simulink model "w13_OOP"  (R2025a)
settings: Solver=VariableStepAuto  StartTime=0.0  StopTime=inf  FixedStep=1e-5  MaxStep=1e-4  RelTol=1e-3
values from neighbouring files (symbols this model uses):
  B = 0.0001    [main.m]
  J = 0.045    [main.m]
  Kic = Rs*Wcc    (= 1256.63706144)    [main.m]
  Kpc = Lds*Wcc    (= 18.8495559215)    [main.m]
  Lamf = 0.12    [main.m]
  Lds = 30.0e-3    (= 0.03)    [main.m]
  Lqs = 40.0e-3    (= 0.04)    [main.m]
  P = 24    [main.m]
  Rs = 2    [main.m]
  V_inj = 60    [main.m]
  w_h = 2*pi*1000    (= 6283.18530718)    [main.m]
settings Model: Creator=moon  LastModifiedBy=mun97
settings RTWCC: GPUComputeCapability=3.5

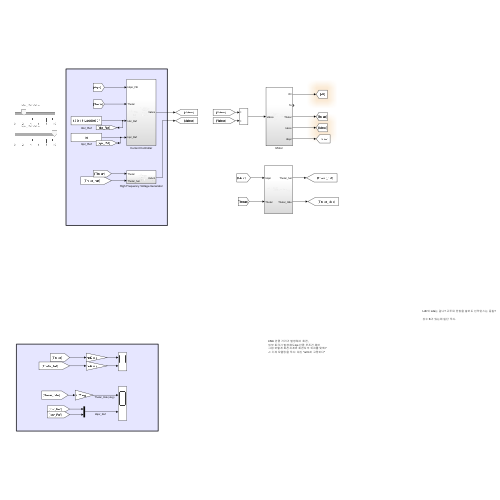
[thumbnail: Simulink's stored preview of the top-level diagram]
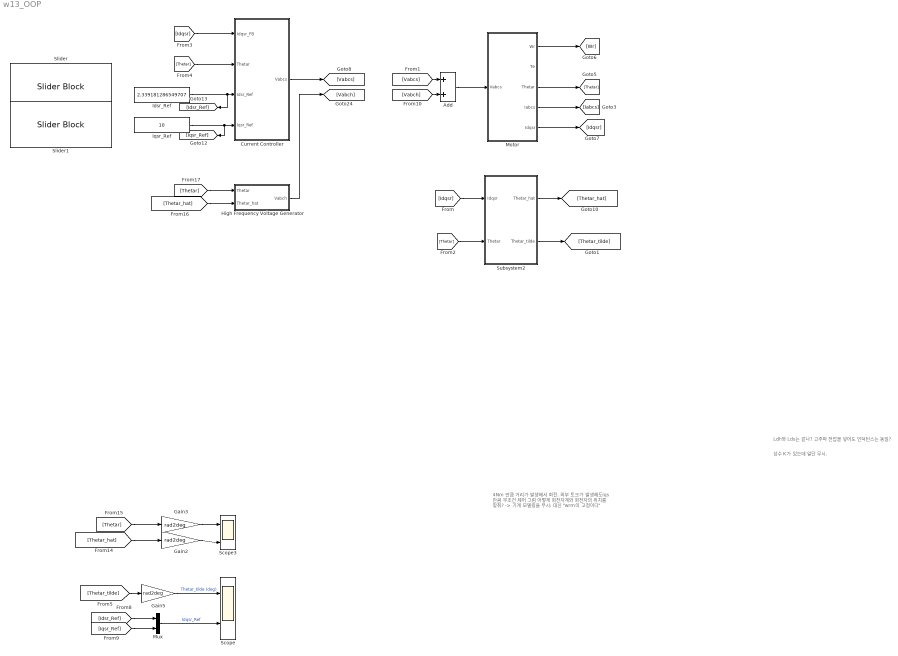
== system w13_OOP ==
  note: Ldh와 Lds는 같나? 고주파 전압을 넣어도 인덕턴스는 동일?
  note: 4Nm 만큼 거리가 발생해서 회전,
      | 외부 토크가 발생해도iqs 만큼 무조건 제어
      | 그럼 어떻게 회전자계와 회전자의 위치를 맞춰?
      | -> 기계 모델링을 무시: 대신 "wrm이 고정이다"
  note: 상수 K가 있는데 일단 무시.
  Add : Sum
  Current Controller : Subsystem
  Gain2 : Gain  Gain=rad2deg
  Gain3 : Gain  Gain=rad2deg
  Gain5 : Gain  Gain=rad2deg
  High Frequency Voltage Generator : Subsystem
  Idsr_Ref : Constant  Value=2.339181286549707
  Iqsr_Ref : Constant  Value=10
  Motor : Subsystem
  Mux : Mux  Inputs=2
  Scope : Scope  NumInputPorts=2
      settings: ActiveDisplayYMinimum=-68.281824450280524  ActiveDisplayYMaximum=129.406425416175  DataLoggingVariableName=ScopeData8
  Scope3 : Scope  NumInputPorts=2
      settings: ActiveDisplayYMinimum=-77.2256556656794  ActiveDisplayYMaximum=78.097651862279335  DataLoggingVariableName=ScopeData11
  Slider : SliderBlock  ScaleMax=10
  Slider1 : SliderBlock  ScaleMax=10
  Subsystem2 : Subsystem
  wires:
  Motor/4(Iabcs) -> [Iabcs]
  Motor/3(Thetar) -> [Thetar]
  Motor/1(Wr) -> [Wr]
  Motor/5(Idqsr) -> [Idqsr]
  [Idqsr] -> Current Controller/1(Idqsr_FB)
  Current Controller/1(Vabcs) -> [Vabcs]
  [Thetar] -> Current Controller/2(Thetar)
  Idsr_Ref/1 -> [Idsr_Ref], Current Controller/3(Idsr_Ref)
  Iqsr_Ref/1 -> Current Controller/4(Iqsr_Ref), [Iqsr_Ref]
  [Vabcs] -> Add/1
  [Vabch] -> Add/2
  Add/1 -> Motor/1(Vabcs)
  [Thetar] -> Gain3/1
  [Thetar_hat] -> Gain2/1
  Gain2/1 -> Scope3/2
  Gain3/1 -> Scope3/1
  Gain5/1 -> Scope/1  "Thetar_tilde (deg)"
  [Thetar_tilde] -> Gain5/1
  [Idsr_Ref] -> Mux/1
  [Iqsr_Ref] -> Mux/2
  Mux/1 -> Scope/2  "Idqsr_Ref"
  High Frequency Voltage Generator/1(Vabch) -> [Vabch]
  [Thetar] -> High Frequency Voltage Generator/1(Thetar)
  [Thetar_hat] -> High Frequency Voltage Generator/2(Thetar_hat)
  [Idqsr] -> Subsystem2/1(Idqsr)
  [Thetar] -> Subsystem2/2(Thetar)
  Subsystem2/1(Thetar_hat) -> [Thetar_hat]
  Subsystem2/2(Thetar_tilde) -> [Thetar_tilde]

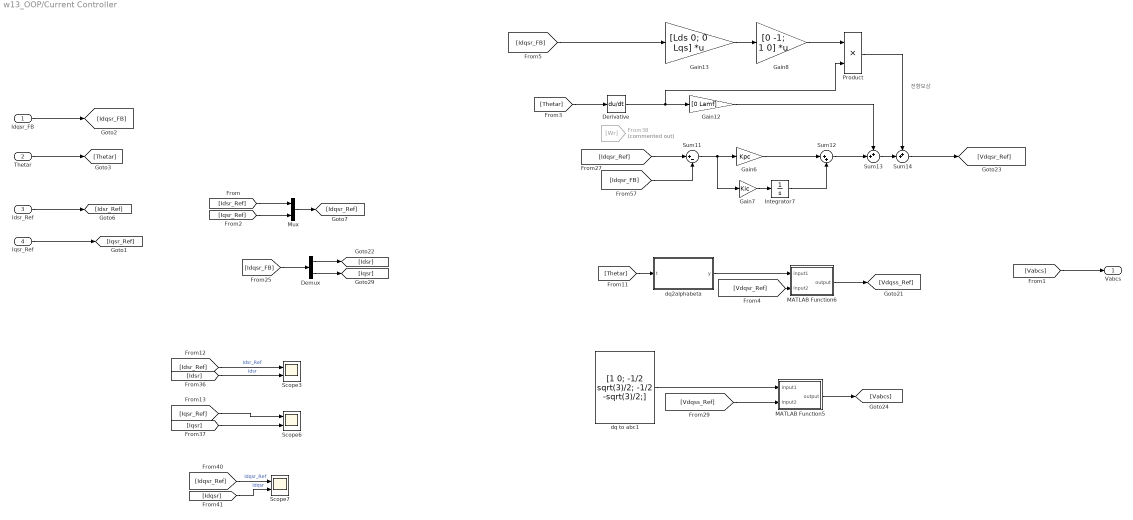
== system w13_OOP/Current Controller ==
  note: 전향보상
  Idqsr_FB : Inport
  Thetar : Inport  Port=2
  Idsr_Ref : Inport  Port=3
  Iqsr_Ref : Inport  Port=4
  Demux : Demux  Outputs=2
  Derivative : Derivative
  From38 : From  Commented=on  GotoTag=Wr
  Gain12 : Gain  Gain=[0 Lamf]
  Gain13 : Gain  Gain=[Lds 0; 0 Lqs]  Multiplication=Matrix(K*u)
  Gain6 : Gain  Gain=Kpc
  Gain7 : Gain  Gain=Kic
  Gain8 : Gain  Gain=[0 -1; 1 0]  Multiplication=Matrix(K*u)
  Integrator7 : Integrator
  MATLAB Function5 : MATLAB Function  TreatAsAtomicUnit=on
  MATLAB Function6 : MATLAB Function  TreatAsAtomicUnit=on
  Mux : Mux  Inputs=2
  Product : Product
  Scope3 : Scope  NumInputPorts=2
      settings: ActiveDisplayYMinimum=-5.30172  ActiveDisplayYMaximum=0.86593  DataLoggingVariableName=ScopeData4
  Scope6 : Scope  NumInputPorts=2
      settings: ActiveDisplayYMinimum=-0.50888  ActiveDisplayYMaximum=4.57994  DataLoggingVariableName=ScopeData5
  Scope7 : Scope  NumInputPorts=2
      settings: ActiveDisplayYMinimum=-5.25048  ActiveDisplayYMaximum=7.25433  DataLoggingVariableName=ScopeData6
  Sum11 : Sum  Inputs=|+-
  Sum12 : Sum  Inputs=|++
  Sum13 : Sum  Inputs=++|
  Sum14 : Sum  Inputs=++|
  dq to abc1 : Constant  Value=[1 0; -1/2 sqrt(3)/2; -1/2 -sqrt(3)/2;]
      mask Display: image(imread('img/dq2abc.png'))
  dq2alphabeta : Subsystem
      mask Display: image(imread('img/rotateMatrix.png'))
  Vabcs : Outport
  wires:
  [Vdqss_Ref] -> MATLAB Function5/2(input2)
  Product/1 -> Sum14/1
  [Thetar] -> dq2alphabeta/1(t)
  [Idqsr] -> Scope7/2  "Idqsr"
  Idsr_Ref/1 -> [Idsr_Ref]
  [Idqsr_FB] -> Gain13/1
  [Iqsr_Ref] -> Scope6/1
  dq2alphabeta/1(y) -> MATLAB Function6/1(input1)
  [Idqsr_Ref] -> Scope7/1  "Idqsr_Ref"
  Demux/2 -> [Iqsr]
  Gain13/1 -> Gain8/1
  [Idsr] -> Scope3/2  "Idsr"
  MATLAB Function6/1(output) -> [Vdqss_Ref]
  Sum14/1 -> [Vdqsr_Ref]
  Sum13/1 -> Sum14/2
  dq to abc1/1 -> MATLAB Function5/1(input1)
  Demux/1 -> [Idsr]
  [Idqsr_FB] -> Sum11/2
  Integrator7/1 -> Sum12/2
  Gain8/1 -> Product/1
  [Idsr_Ref] -> Scope3/1  "Idsr_Ref"
  Gain6/1 -> Sum12/1
  Derivative/1 -> Product/2, Gain12/1
  [Idqsr_Ref] -> Sum11/1
  MATLAB Function5/1(output) -> [Vabcs]
  [Iqsr] -> Scope6/2
  Gain12/1 -> Sum13/1
  [Idqsr_FB] -> Demux/1
  Sum11/1 -> Gain7/1, Gain6/1
  [Vdqsr_Ref] -> MATLAB Function6/2(input2)
  Sum12/1 -> Sum13/2
  Gain7/1 -> Integrator7/1
  Idqsr_FB/1 -> [Idqsr_FB]
  [Vabcs] -> Vabcs/1
  Thetar/1 -> [Thetar]
  Iqsr_Ref/1 -> [Iqsr_Ref]
  [Idsr_Ref] -> Mux/1
  Mux/1 -> [Idqsr_Ref]
  [Iqsr_Ref] -> Mux/2
  [Thetar] -> Derivative/1

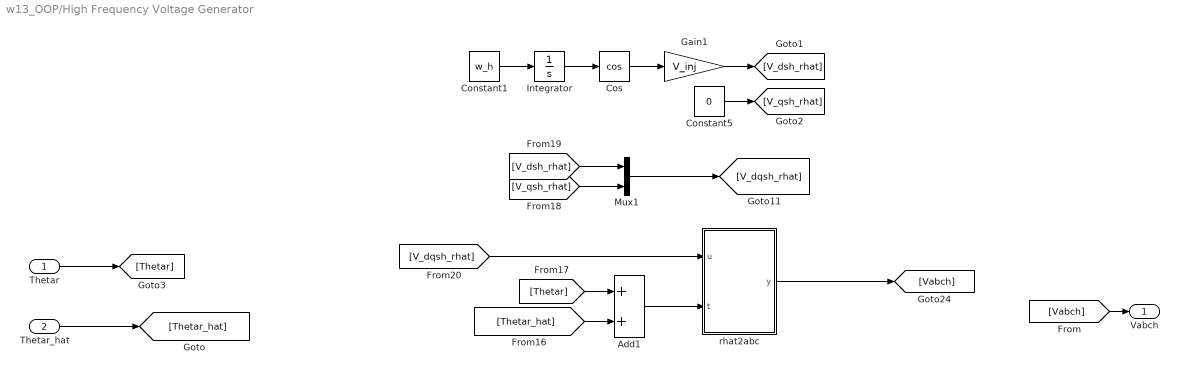
== system w13_OOP/High Frequency Voltage Generator ==
  Thetar : Inport
  Thetar_hat : Inport  Port=2
  Add1 : Sum
  Constant1 : Constant  Value=w_h
  Constant5 : Constant  Value=0
  Cos : Trigonometry  Operator=cos
  Gain1 : Gain  Gain=V_inj
  Integrator : Integrator
  Mux1 : Mux  Inputs=2
  rhat2abc : MATLAB Function  TreatAsAtomicUnit=on
  Vabch : Outport
  wires:
  Constant5/1 -> [V_qsh_rhat]
  Integrator/1 -> Cos/1
  Constant1/1 -> Integrator/1
  Mux1/1 -> [V_dqsh_rhat]
  Gain1/1 -> [V_dsh_rhat]
  rhat2abc/1(y) -> [Vabch]
  Add1/1 -> rhat2abc/2(t)
  Cos/1 -> Gain1/1
  [V_dsh_rhat] -> Mux1/1
  [V_qsh_rhat] -> Mux1/2
  [Thetar_hat] -> Add1/2
  [Thetar] -> Add1/1
  [V_dqsh_rhat] -> rhat2abc/1(u)
  [Vabch] -> Vabch/1
  Thetar_hat/1 -> [Thetar_hat]
  Thetar/1 -> [Thetar]

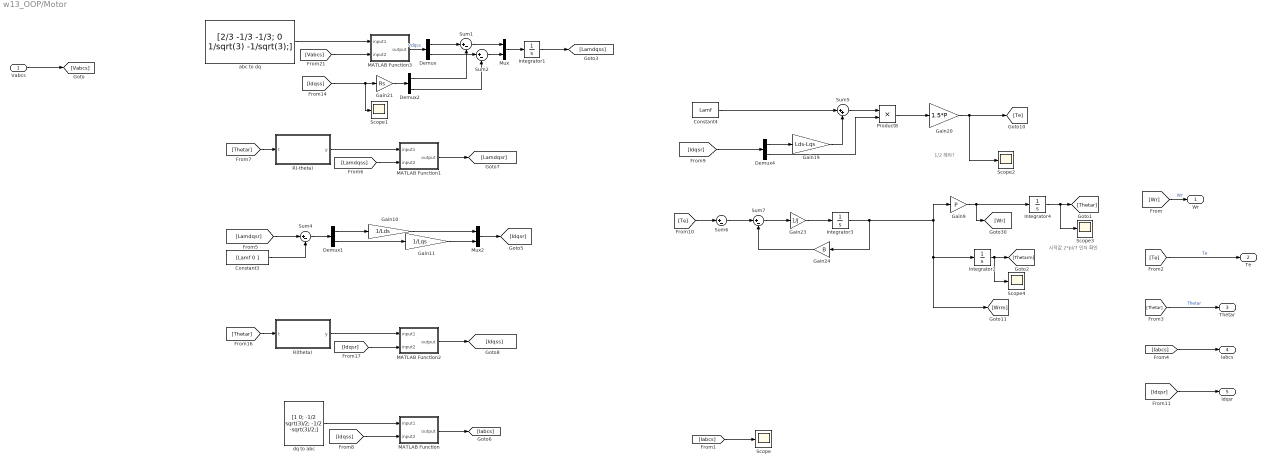
== system w13_OOP/Motor ==
  note: 시작값 2*pi/7 인지 확인
  note: 1/2 해야?
  Vabcs : Inport
  Constant3 : Constant  Value=[Lamf 0 ]
  Constant4 : Constant  Value=Lamf
  Demux{,1..2,4} (4 alike) : Demux  Outputs=2
  Gain10 : Gain  Gain=1/Lds
  Gain11 : Gain  Gain=1/Lqs
  Gain19 : Gain  Gain=Lds-Lqs
  Gain20 : Gain  Gain=1.5*P
  Gain21 : Gain  Gain=Rs
  Gain23 : Gain  Gain=1/J
  Gain24 : Gain  Gain=B
  Gain9 : Gain  Gain=P
  Integrator1 : Integrator
  Integrator2 : Integrator
  Integrator3 : Integrator
  Integrator4 : Integrator  InitialCondition=pi/4
  MATLAB Function : MATLAB Function  TreatAsAtomicUnit=on
  MATLAB Function1 : MATLAB Function  TreatAsAtomicUnit=on
  MATLAB Function2 : MATLAB Function  TreatAsAtomicUnit=on
  MATLAB Function3 : MATLAB Function  TreatAsAtomicUnit=on
  Mux : Mux  Inputs=2
  Mux2 : Mux  Inputs=2
  Product8 : Product
  R(-theta) : Subsystem
      mask Display: image(imread('img/rotateInverseMatrix.png'))
  R(theta) : Subsystem
      mask Display: image(imread('img/rotateMatrix.png'))
  Scope{,1..4} (5 alike) : Scope
      Scope settings: ActiveDisplayYMinimum=-12.65498  ActiveDisplayYMaximum=12.66704
      Scope1 settings: ActiveDisplayYMinimum=-1  ActiveDisplayYMaximum=1
      Scope2 settings: ActiveDisplayYMinimum=-25.248088739703935  ActiveDisplayYMaximum=48.434171321935082  DataLoggingVariableName=ScopeData2
      Scope3 settings: ActiveDisplayYMinimum=-29.096358218238635  ActiveDisplayYMaximum=1.9302061013316951  DataLoggingVariableName=ScopeData7
      Scope4 settings: ActiveDisplayYMinimum=-0.083156272772802617  ActiveDisplayYMaximum=0.00891129758026395  DataLoggingVariableName=ScopeData12
  Sum{1..2,4,6..7} (5 alike) : Sum  Inputs=|+-
  Sum5 : Sum  Inputs=|++
  abc to dq : Constant  Value=[2/3 -1/3 -1/3; 0 1/sqrt(3) -1/sqrt(3);]
      mask Display: image(imread('img/abc2dq.png'))
  dq to abc : Constant  Value=[1 0; -1/2 sqrt(3)/2; -1/2 -sqrt(3)/2;]
      mask Display: image(imread('img/dq2abc.png'))
  Wr : Outport
  Te : Outport  Port=2
  Thetar : Outport  Port=3
  Iabcs : Outport  Port=4
  Idqsr : Outport  Port=5
  wires:
  R(-theta)/1(y) -> MATLAB Function1/1(input1)
  [Idqsr] -> Demux4/1
  Product8/1 -> Gain20/1
  Sum7/1 -> Gain23/1
  Sum5/1 -> Product8/1
  [Thetar] -> R(theta)/1(t)
  [Lamdqsr] -> Sum4/1
  [Idqss] -> Scope1/1, Gain21/1
  R(theta)/1(y) -> MATLAB Function2/1(input1)
  Gain24/1 -> Sum7/2
  MATLAB Function/1(output) -> [Iabcs]
  Constant4/1 -> Sum5/1
  [Thetar] -> R(-theta)/1(t)
  MATLAB Function2/1(output) -> [Idqss]
  [Vabcs] -> MATLAB Function3/2(input2)
  Demux1/2 -> Gain11/1
  abc to dq/1 -> MATLAB Function3/1(input1)
  Gain20/1 -> Scope2/1, [Te]
  Integrator1/1 -> [Lamdqss]
  [Iabcs] -> Scope/1
  [Idqsr] -> MATLAB Function2/2(input2)
  Gain23/1 -> Integrator3/1
  Demux1/1 -> Gain10/1
  [Idqss] -> MATLAB Function/2(input2)
  Gain19/1 -> Sum5/2
  dq to abc/1 -> MATLAB Function/1(input1)
  Gain11/1 -> Mux2/2
  Demux4/2 -> Product8/2
  MATLAB Function1/1(output) -> [Lamdqsr]
  Mux2/1 -> [Idqsr]
  Constant3/1 -> Sum4/2
  Gain10/1 -> Mux2/1
  [Te] -> Sum6/1
  Integrator3/1 -> Gain24/1, Integrator2/1, [Wrm], Gain9/1
  Sum6/1 -> Sum7/1
  [Lamdqss] -> MATLAB Function1/2(input2)
  Sum4/1 -> Demux1/1
  Demux4/1 -> Gain19/1
  Vabcs/1 -> [Vabcs]
  [Wr] -> Wr/1  "Wr"
  [Te] -> Te/1  "Te"
  [Thetar] -> Thetar/1  "Thetar"
  [Iabcs] -> Iabcs/1
  [Idqsr] -> Idqsr/1
  MATLAB Function3/1(output) -> Demux/1  "Vdqss"
  Gain21/1 -> Demux2/1
  Sum2/1 -> Mux/2
  Sum1/1 -> Mux/1
  Demux2/1 -> Sum1/2
  Demux2/2 -> Sum2/2
  Demux/2 -> Sum2/1
  Demux/1 -> Sum1/1
  Mux/1 -> Integrator1/1
  Gain9/1 -> [Wr], Integrator4/1
  Integrator4/1 -> Scope3/1, [Thetar]
  Integrator2/1 -> Scope4/1, [Thetarm]

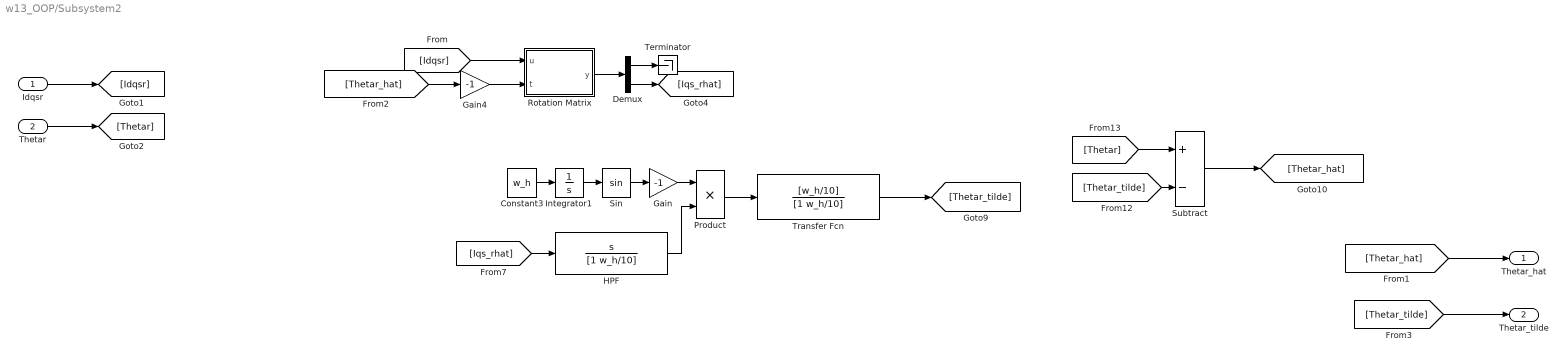
== system w13_OOP/Subsystem2 ==
  Idqsr : Inport
  Thetar : Inport  Port=2
  Constant3 : Constant  Value=w_h
  Demux : Demux  Outputs=2
  Gain : Gain  Gain=-1
  Gain4 : Gain  Gain=-1
  HPF : TransferFcn  Numerator=[1 0]  Denominator=[1 w_h/10]
  Integrator1 : Integrator
  Product : Product
  Rotation Matrix : MATLAB Function  TreatAsAtomicUnit=on
  Sin : Trigonometry
  Subtract : Sum  Inputs=+-
  Terminator : Terminator
  Transfer Fcn : TransferFcn  Numerator=[w_h/10]  Denominator=[1 w_h/10]
  Thetar_hat : Outport
  Thetar_tilde : Outport  Port=2
  wires:
  Subtract/1 -> [Thetar_hat]
  Product/1 -> Transfer Fcn/1
  Constant3/1 -> Integrator1/1
  Demux/2 -> [Iqs_rhat]
  Rotation Matrix/1(y) -> Demux/1
  Gain4/1 -> Rotation Matrix/2(t)
  [Iqs_rhat] -> HPF/1
  Integrator1/1 -> Sin/1
  HPF/1 -> Product/2
  [Thetar_tilde] -> Subtract/2
  Transfer Fcn/1 -> [Thetar_tilde]
  Demux/1 -> Terminator/1
  [Thetar] -> Subtract/1
  Sin/1 -> Gain/1
  [Thetar_hat] -> Gain4/1
  [Idqsr] -> Rotation Matrix/1(u)
  Idqsr/1 -> [Idqsr]
  Thetar/1 -> [Thetar]
  [Thetar_hat] -> Thetar_hat/1
  Gain/1 -> Product/1
  [Thetar_tilde] -> Thetar_tilde/1

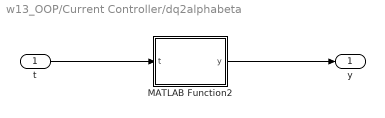
== system w13_OOP/Current Controller/dq2alphabeta ==
  t : Inport
  MATLAB Function2 : MATLAB Function  TreatAsAtomicUnit=on
  y : Outport
  wires:
  MATLAB Function2/1(y) -> y/1
  t/1 -> MATLAB Function2/1(t)

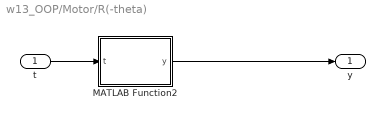
== system w13_OOP/Motor/R(-theta) ==
  t : Inport
  MATLAB Function2 : MATLAB Function  TreatAsAtomicUnit=on
  y : Outport
  wires:
  MATLAB Function2/1(y) -> y/1
  t/1 -> MATLAB Function2/1(t)

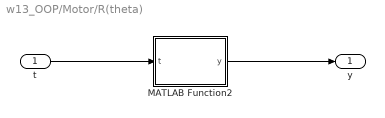
== system w13_OOP/Motor/R(theta) ==
  t : Inport
  MATLAB Function2 : MATLAB Function  TreatAsAtomicUnit=on
  y : Outport
  wires:
  MATLAB Function2/1(y) -> y/1
  t/1 -> MATLAB Function2/1(t)

== matlab function w13_OOP/Motor/MATLAB Function ==
  data: input1 input; output output; input2 input
function output = matrix_multiply(input1, input2)
    % 행렬 곱셈 (input1의 열 수 = input2의 행 수)
    output = input1 * input2;
end

== matlab function w13_OOP/Motor/R(-theta)/MATLAB Function2 ==
  data: t input; y output
function y = matrix_output(t)
y = [cos(t) sin(t); -sin(t) cos(t)];

== matlab function w13_OOP/Motor/MATLAB Function2 ==
  data: input1 input; output output; input2 input
function output = matrix_multiply(input1, input2)
    % 행렬 곱셈 (input1의 열 수 = input2의 행 수)
    output = input1 * input2;
end

== matlab function w13_OOP/Motor/R(theta)/MATLAB Function2 ==
  data: t input; y output
function y = matrix_output(t)
y = [cos(t) -sin(t); sin(t) cos(t)];

== matlab function w13_OOP/Motor/MATLAB Function3 ==
  data: input1 input; output output; input2 input size=[3 1]
function output = matrix_multiply(input1, input2)
    % 행렬 곱셈 (input1의 열 수 = input2의 행 수)
    output = input1 * input2;
end

== matlab function w13_OOP/Subsystem2/Rotation Matrix ==
  data: u input size=[2 1]; y output size=[2 1]; t input
function y = fcn(u, t)

R = [cos(t) -sin(t); sin(t) cos(t)];

y = R*u;

== matlab function w13_OOP/Current Controller/MATLAB Function5 ==
  data: input1 input; output output; input2 input
function output = matrix_multiply(input1, input2)
    % 행렬 곱셈 (input1의 열 수 = input2의 행 수)
    output = input1 * input2;
end

== matlab function w13_OOP/Current Controller/MATLAB Function6 ==
  data: input1 input; output output; input2 input
function output = matrix_multiply(input1, input2)
    % 행렬 곱셈 (input1의 열 수 = input2의 행 수)
    output = input1 * input2;
end

== matlab function w13_OOP/Current Controller/dq2alphabeta/MATLAB Function2 ==
  data: t input; y output
function y = matrix_output(t)
y = [cos(t) -sin(t); sin(t) cos(t)];

== matlab function w13_OOP/Motor/MATLAB Function1 ==
  data: input1 input; output output; input2 input
function output = matrix_multiply(input1, input2)
    % 행렬 곱셈 (input1의 열 수 = input2의 행 수)
    output = input1 * input2;
end

== matlab function w13_OOP/High Frequency Voltage Generator/rhat2abc ==
  data: u input size=[2 1]; y output size=[3 1]; t input
function y = fcn(u, t)

a=2*pi/3;

TT = @(t) ...
    [cos(t)  cos(t-a)  cos(t+a);
    -sin(t) -sin(t-a) -sin(t+a);
        1/2       1/2       1/2;] *2/3;

y = TT(t) \ [u; 0];
